simulink subsystem "pam_tx"  (R2019b)
settings: Solver=VariableStepAuto  StartTime=0.0  StopTime=10.0  RelTol=1e-3
libraries: commutil2 x2, commdigbbndam3 x1, commrandsrc3 x1
settings Model: Creator=yango  LastModifiedBy=yango

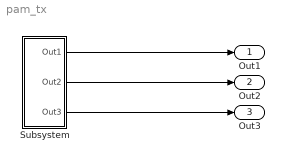
== system pam_tx ==
  Subsystem : Subsystem
  Out1 : Outport  SignalName=Bit
  Out2 : Outport  Port=2  SignalName=Symbol
  Out3 : Outport  Port=3  SignalName=Modulated Signal
  wires:
  Subsystem/1(Out1) -> Out1/1
  Subsystem/2(Out2) -> Out2/1
  Subsystem/3(Out3) -> Out3/1

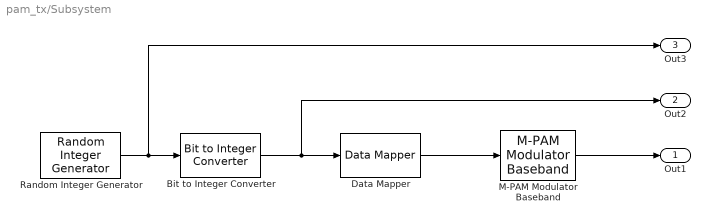
== system pam_tx/Subsystem ==
  Bit to Integer Converter : commutil2/Bit to Integer Converter  nbits=2  bitOrder=MSB first  signedOutputValues=Unsigned  outDtype=Inherit via internal rule  outDtypeSigned=Inherit via internal rule
      settings: SourceProductName=Communications Toolbox
  Data Mapper : commutil2/Data Mapper  MapMode=Binary to Gray  M=4  MapVec=[0 1 3 2 7 6 4 5]
      settings: SourceProductName=Communications Toolbox  SourceProductBaseCode=CM
  M-PAM Modulator Baseband : commdigbbndam3/M-PAM Modulator Baseband  M=4  InType=Integer  Enc=Gray  PowType=Min. distance between symbols  MinDist=2  AvgPow=1  PeakPow=1  outDtype=double  outWordLen=16  outUDDataType=sfix(16)  outFracLenMode=Best precision  outFracLen=15  outDataTypeStr=double  outLastDataTypeStr=double
      settings: SourceProductName=Communications Toolbox  SourceProductBaseCode=CM
  Random Integer Generator : commrandsrc3/Random Integer Generator  SetSize=2  SeedSource=Auto  Seed=0  SampleTime=1/200000  SamplesPerFrame=200000  OutputDataType=double  SimulateUsing=Interpreted execution
      settings: SourceProductName=Communications Toolbox
  Out1 : Outport
  Out2 : Outport  Port=2
  Out3 : Outport  Port=3
  wires:
  Bit to Integer Converter/1 -> Out2/1, Data Mapper/1
  M-PAM Modulator Baseband/1 -> Out1/1
  Random Integer Generator/1 -> Out3/1, Bit to Integer Converter/1
  Data Mapper/1 -> M-PAM Modulator Baseband/1
